simulink model "ProjetoRosely"  (Simulink 7.4)
settings: Solver=ode45  StartTime=0.0  StopTime=10.0  RelTol=1e-3
values from neighbouring files (symbols this model uses):
  B = 0.0078    [trabalhoautomacao_TP1.m]
  J = 3.79    [trabalhoautomacao_TP1.m]
  k3 = 12.8    [trabalhoautomacao_TP1.m]
  kb = 1.28    [trabalhoautomacao_TP1.m]
  La = 1111111111.043    (= 1111111111.04)    [trabalhoautomacao_TP1.m]
  Ra = 2.4    [trabalhoautomacao_TP1.m]
settings Model: Creator=Fabiano  LastModifiedBy=Fabiano

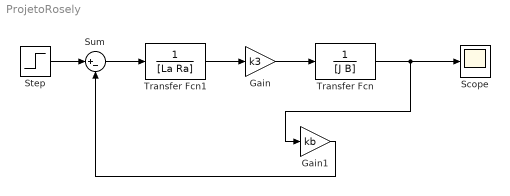
== system ProjetoRosely ==
  Gain : Gain  Gain=k3  ParameterDataType=fixdt(1, 16)  ParameterScaling=2^0  OutDataType=fixdt(1, 16)  OutScaling=2^0
  Gain1 : Gain  Gain=kb  ParameterDataType=fixdt(1, 16)  ParameterScaling=2^0  OutDataType=fixdt(1, 16)  OutScaling=2^0
  Scope : Scope
  Step : Step  After=220  SampleTime=0
  Sum : Sum  Inputs=|+-  OutDataType=fixdt(1, 16)  OutScaling=2^0
  Transfer Fcn : TransferFcn  Denominator=[J B]
  Transfer Fcn1 : TransferFcn  Denominator=[La Ra]
  wires:
  Sum/1 -> Transfer Fcn1/1
  Transfer Fcn1/1 -> Gain/1
  Gain/1 -> Transfer Fcn/1
  Transfer Fcn/1 -> Scope/1, Gain1/1
  Gain1/1 -> Sum/2
  Step/1 -> Sum/1
